simulink model "second_cl"  (R2019b)
settings: Solver=VariableStepAuto  StartTime=0.0  StopTime=10  RelTol=1e-3
values from neighbouring files (symbols this model uses):
  K = lqr_controller(sys)    [ex3main.m]
  Ts = 1/200    (= 0.005)    [ex3main.m]
  wc = 2*f*pi    (= 12.5663706144)    [ex3main.m]
  x_d = desired_state(theta_d, params)    [ex3main.m]
undefined symbols (not defined in the file or in its folder): sys2
settings Model: Creator=martijndebeuf  LastModifiedBy=martijndebeuf

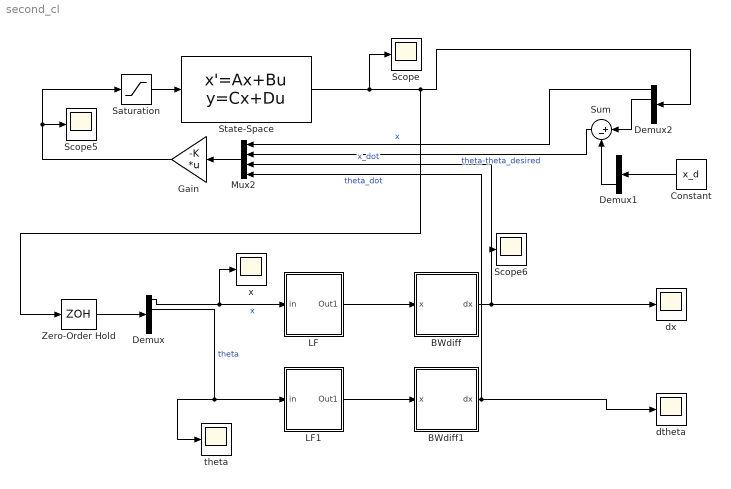
== system second_cl ==
  BWdiff : Subsystem
  BWdiff1 : Subsystem
  Constant : Constant  Value=x_d
  Demux : Demux
  Demux1 : Demux  Outputs=2
  Demux2 : Demux
  Gain : Gain  Gain=-K  Multiplication=Matrix(K*u) (u vector)
  LF : Subsystem
  LF1 : Subsystem
  Mux2 : Mux
  Saturation : Saturate  UpperLimit=5  LowerLimit=-5
  Scope : Scope
  Scope5 : Scope
  Scope6 : Scope
  State-Space : StateSpace  A=sys2.A  B=sys2.B  C=eye(4)  D=zeros(4,1)  InitialCondition=initial_conditions'
  Sum : Sum  Inputs=|+-
  Zero-Order Hold : ZeroOrderHold  SampleTime=Ts
  dtheta : Scope
  dx : Scope
  theta : Scope
  x : Scope
  wires:
  Demux/1 -> LF/1(in), x/1  "x"
  Demux/2 -> LF1/1(in), theta/1  "theta"
  BWdiff/1(dx) -> Mux2/3, Scope6/1, dx/1  "x_dot"
  BWdiff1/1(dx) -> Mux2/4, dtheta/1  "theta_dot"
  Saturation/1 -> State-Space/1
  Mux2/1 -> Gain/1
  Constant/1 -> Demux1/1
  Demux1/2 -> Sum/2
  Demux2/2 -> Sum/1
  Sum/1 -> Mux2/2  "theta-theta_desired"
  Demux2/1 -> Mux2/1  "x"
  State-Space/1 -> Scope/1, Zero-Order Hold/1, Demux2/1
  Gain/1 -> Scope5/1, Saturation/1
  LF/1(Out1) -> BWdiff/1(x)
  LF1/1(Out1) -> BWdiff1/1(x)
  Zero-Order Hold/1 -> Demux/1

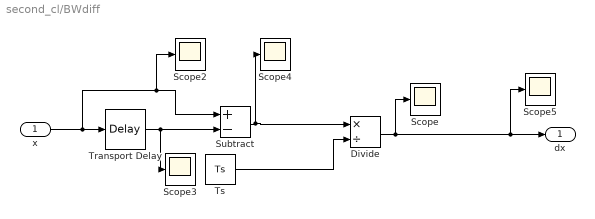
== system second_cl/BWdiff ==
  x : Inport
  Divide : Product  Inputs=*/
  Scope{,2..5} (5 alike) : Scope
  Subtract : Sum  Inputs=+-
  Transport Delay : TransportDelay  DelayTime=Ts
  Ts : Constant  Value=Ts
  dx : Outport
  wires:
  Transport Delay/1 -> Scope3/1, Subtract/2
  Ts/1 -> Divide/2
  x/1 -> Transport Delay/1, Scope2/1, Subtract/1
  Subtract/1 -> Divide/1, Scope4/1
  Divide/1 -> Scope5/1, dx/1, Scope/1

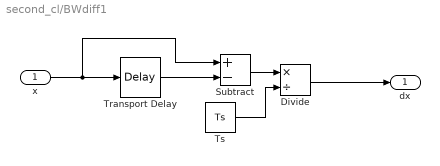
== system second_cl/BWdiff1 ==
  x : Inport
  Divide : Product  Inputs=*/
  Subtract : Sum  Inputs=+-
  Transport Delay : TransportDelay  DelayTime=Ts
  Ts : Constant  Value=Ts
  dx : Outport
  wires:
  Ts/1 -> Divide/2
  Subtract/1 -> Divide/1
  x/1 -> Transport Delay/1, Subtract/1
  Divide/1 -> dx/1
  Transport Delay/1 -> Subtract/2

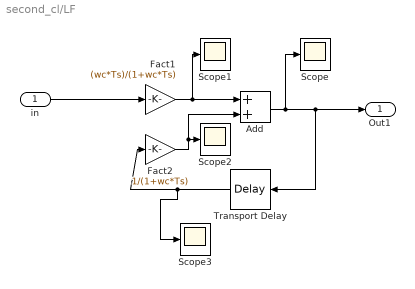
== system second_cl/LF ==
  in : Inport
  Add : Sum
  Fact1 : Gain  Gain=(wc*Ts)/(1+wc*Ts)
  Fact2 : Gain  Gain=1/(1+wc*Ts)
  Scope{,1..3} (4 alike) : Scope
  Transport Delay : TransportDelay  DelayTime=Ts
  Out1 : Outport
  wires:
  Fact2/1 -> Add/2, Scope2/1
  Fact1/1 -> Scope1/1, Add/1
  in/1 -> Fact1/1
  Add/1 -> Scope/1, Transport Delay/1, Out1/1
  Transport Delay/1 -> Scope3/1, Fact2/1

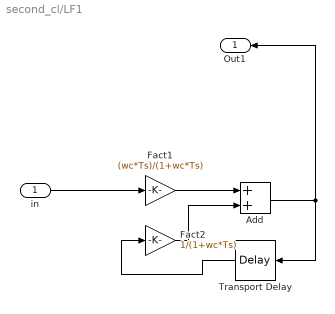
== system second_cl/LF1 ==
  in : Inport
  Add : Sum
  Fact1 : Gain  Gain=(wc*Ts)/(1+wc*Ts)
  Fact2 : Gain  Gain=1/(1+wc*Ts)
  Transport Delay : TransportDelay  DelayTime=Ts
  Out1 : Outport
  wires:
  Add/1 -> Transport Delay/1, Out1/1
  Fact2/1 -> Add/2
  Fact1/1 -> Add/1
  in/1 -> Fact1/1
  Transport Delay/1 -> Fact2/1
